simulink model "MultiSiteCoherenceTriggerDetector"  (R2016b)
settings: Solver=FixedStepDiscrete  StartTime=0.0  StopTime=inf  FixedStep=sCoreParams.core.stepPeriod  RelTol=1e-3
undefined symbols (not defined in the file): Low, sCoreParams, sCoreParams_decoders_txDetector_anyAll, sCoreParams_decoders_txDetector_detectChannelInds, sCoreParams_decoders_txDetector_nDetectionsRequested, sCoreParams_decoders_txDetector_ProbabilityOfStim, sCoreParams_decoders_txDetector_txRMS, sCoreParams_decoders_txDetector_txRMSLower, sCoreParams_decoders_txDetector_txSign, sCoreParams_stimulator_possibleStimRealChannelNumbers
libraries: simulink x3, dspswit3 x3, dspsigops x1
settings Model: DataTypeOverride=Double  MinMaxOverflowLogging=ForceOff  ParamWorkspaceSource=ReferencedWorkspace  Creator=anish  LastModifiedBy=rzelmann
settings SolverCC: EnableConcurrentExecution=on
settings DataIOCC: SaveFormat=StructureWithTime  SignalLoggingSaveFormat=ModelDataLogs  SaveOutput=off  SignalLogging=off  DSMLogging=off  SaveTime=off
settings OptimizationCC: BlockReduction=off  ConditionallyExecuteInputs=off  DefaultParameterBehavior=Inlined  OptimizeBlockIOStorage=off  BufferReuse=off  GlobalBufferReuse=off  ExpressionFolding=off  LocalBlockOutputs=off  LifeSpan=inf
settings DebuggingCC: SignalRangeChecking=error  SaveWithParameterizedLinksMsg=none  MultiTaskDSMMsg=warning  MultiTaskCondExecSysMsg=none  AllowSymbolicDim=off  ModelReferenceSymbolNameMessage=none  StateNameClashWarn=warning  SFUnexpectedBacktrackingDiag=warning  SFNoUnconditionalDefaultTransitionDiag=warning  SFExecutionAtInitializationDiag=none
settings HardwareCC: ProdBitPerPointer=32  ProdBitPerSizeT=32  ProdBitPerPtrDiffT=32  ProdLargestAtomicFloat=None  ProdWordSize=32  ProdLongLongMode=on  ProdHWDeviceType=Generic->32-bit x86 compatible  TargetBitPerPointer=64  TargetLargestAtomicFloat=Float  TargetLongLongMode=on  TargetIntDivRoundTo=Zero  TargetEndianess=LittleEndian  TargetWordSize=64  TargetHWDeviceType=Intel->x86-64 (Windows64)
settings ModelReferenceCC: ModelReferenceNumInstancesAllowed=Single  ModelReferencePassRootInputsByReference=off
settings RTWCC: SystemTargetFile=slrt.tlc  TemplateMakefile=slrt_default_tmf  Description=Simulink Real-Time  BuildConfiguration=Faster Runs  RTWCompilerOptimization=on
settings ConfigComp: CovMetricSettings=dw  CovHtmlReporting=on  CovSaveCumulativeToWorkspaceVar=on  CovSaveSingleToWorkspaceVar=on  CovExternalEMLEnable=off  CovSFcnEnable=off

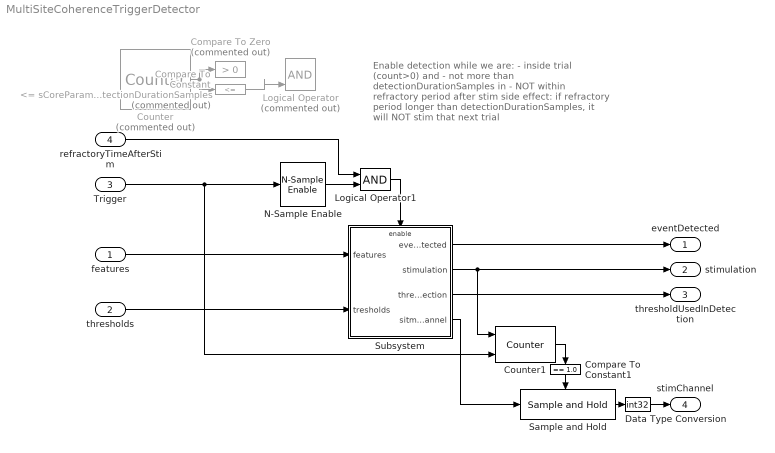
== system MultiSiteCoherenceTriggerDetector ==
  note: Enable detection while we are:
      |  -  inside trial (count>0) and
      | - not more than detectionDurationSamples in
      | - NOT within refractory period after stim
      | side effect: if refractory period longer than detectionDurationSamples, it will NOT stim that next trial
  features : Inport  PortDimensions=[1 sCoreParams.decoders.txDetector.nPairs]  SampleTime=sCoreParams.core.stepPeriod
  thresholds : Inport  Port=2  PortDimensions=[1 sCoreParams.decoders.txDetector.nPairs]  SampleTime=sCoreParams.core.stepPeriod
  Trigger : Inport  Port=3  OutDataTypeStr=int32
  refractoryTimeAfterStim : Inport  Port=4  OutDataTypeStr=boolean  SampleTime=sCoreParams.core.stepPeriod
  Compare To Constant : simulink/Logic and Bit Operations/Compare To Constant  Commented=on  relop=<=  const=sCoreParams.decoders.txDetector.detectionDurationSamples  OutDataTypeStr=boolean
  Compare To Constant1 : simulink/Logic and Bit Operations/Compare To Constant  relop===  const=1.0  OutDataTypeStr=boolean
  Compare To Zero : simulink/Logic and Bit Operations/Compare To Zero  Commented=on  relop=>  OutDataTypeStr=boolean
  Counter : dspswit3/Counter  Commented=on  Direction=Up  CountEvent=Free running  CounterSize=16 bits  MaxCount=255  InitialCount=0  Output=Count  HitValue=sCoreParams.decoders.txDetector.detectionDurationSamples  ResetInput=on  SamplesPerFrame=1  Ts=sCoreParams.core.stepPeriod  CntDtype=int32  HitDtype=Logical
  Counter1 : dspswit3/Counter  Direction=Up  CountEvent=Rising edge  CounterSize=User defined  MaxCount=1024  InitialCount=0  Output=Count  HitValue=1  ResetInput=on  SamplesPerFrame=1  Ts=1  CntDtype=double  HitDtype=Logical
  Data Type Conversion : DataTypeConversion  OutDataTypeStr=int32
  Logical Operator : Logic  Commented=on  IconShape=distinctive  AllPortsSameDT=off  OutDataTypeStr=boolean
  Logical Operator1 : Logic  IconShape=distinctive  AllPortsSameDT=off  OutDataTypeStr=boolean
  N-Sample Enable : dspswit3/N-Sample Enable  N=sCoreParams.decoders.txDetector.detectionDurationSamples  ActiveLevel=Low (0)  reset=on  TriggerType=Non-zero sample  Ts=1  DataType=Logical
  Sample and Hold : dspsigops/Sample and Hold  trig=Rising edge  initCond=0  latchinput=off
  Subsystem : Subsystem
  eventDetected : Outport  SampleTime=sCoreParams.core.stepPeriod
  stimulation : Outport  Port=2  SampleTime=sCoreParams.core.stepPeriod
  thresholdUsedInDetection : Outport  Port=3  SampleTime=sCoreParams.core.stepPeriod
  stimChannel : Outport  Port=4  OutDataTypeStr=int32
  wires:
  features/1 -> Subsystem/1(features)
  thresholds/1 -> Subsystem/2(tresholds)
  Subsystem/1(eventDetected) -> eventDetected/1
  Subsystem/2(stimulation) -> stimulation/1, Counter1/1
  Subsystem/3(thresholdUsedInDetection) -> thresholdUsedInDetection/1
  Trigger/1 -> Counter1/2, N-Sample Enable/1
  Logical Operator1/1 -> Subsystem/Enable
  Subsystem/4(sitmChannel) -> Sample and Hold/1
  Data Type Conversion/1 -> stimChannel/1
  Counter/1 -> Compare To Constant/1, Compare To Zero/1
  Compare To Constant/1 -> Logical Operator/2
  Sample and Hold/1 -> Data Type Conversion/1
  Counter1/1 -> Compare To Constant1/1
  refractoryTimeAfterStim/1 -> Logical Operator1/1
  N-Sample Enable/1 -> Logical Operator1/2
  Compare To Constant1/1 -> Sample and Hold/Trigger

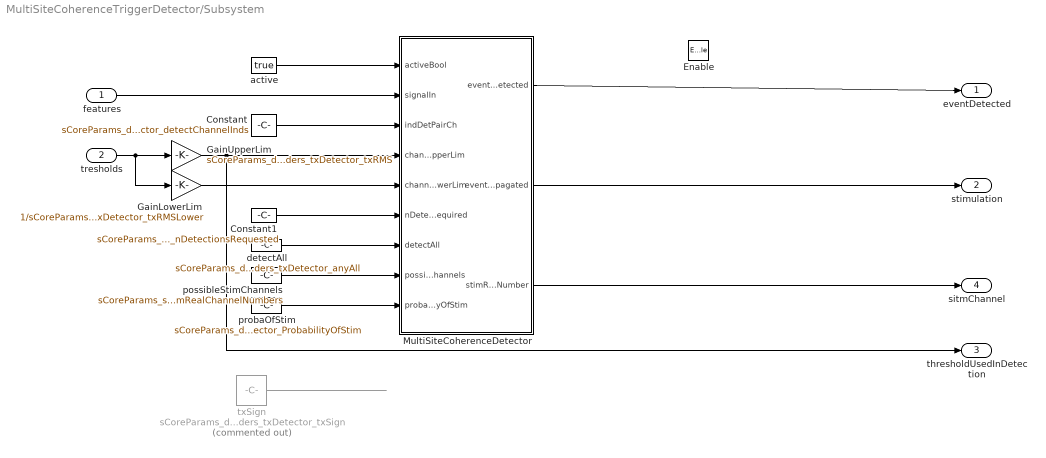
== system MultiSiteCoherenceTriggerDetector/Subsystem ==
  features : Inport
  tresholds : Inport  Port=2
  Enable : EnablePort
  Constant : Constant  Value=sCoreParams_decoders_txDetector_detectChannelInds  SampleTime=Inf
  Constant1 : Constant  Value=sCoreParams_decoders_txDetector_nDetectionsRequested  SampleTime=Inf
  GainLowerLim : Gain  Gain=1/sCoreParams_decoders_txDetector_txRMSLower
  GainUpperLim : Gain  Gain=sCoreParams_decoders_txDetector_txRMS
  MultiSiteCoherenceDetector : MATLAB Function  TreatAsAtomicUnit=on
  active : Constant  Value=true
  detectAll : Constant  Value=sCoreParams_decoders_txDetector_anyAll
  possibleStimChannels : Constant  Value=sCoreParams_stimulator_possibleStimRealChannelNumbers
  probaOfStim : Constant  Value=sCoreParams_decoders_txDetector_ProbabilityOfStim
  txSign : Constant  Commented=on  Value=sCoreParams_decoders_txDetector_txSign
  eventDetected : Outport
  stimulation : Outport  Port=2
  thresholdUsedInDetection : Outport  Port=3
  sitmChannel : Outport  Port=4
  wires:
  GainUpperLim/1 -> thresholdUsedInDetection/1, MultiSiteCoherenceDetector/4(channelThresholdUpperLim)
  MultiSiteCoherenceDetector/2(eventPropagated) -> stimulation/1
  Constant/1 -> MultiSiteCoherenceDetector/3(indDetPairCh)
  Constant1/1 -> MultiSiteCoherenceDetector/6(nDetectionsRequired)
  active/1 -> MultiSiteCoherenceDetector/1(activeBool)
  txSign/1 -> ?
  features/1 -> MultiSiteCoherenceDetector/2(signalIn)
  MultiSiteCoherenceDetector/1(eventDetected) -> eventDetected/1
  tresholds/1 -> GainLowerLim/1, GainUpperLim/1
  detectAll/1 -> MultiSiteCoherenceDetector/7(detectAll)
  MultiSiteCoherenceDetector/3(stimRealChannelNumber) -> sitmChannel/1
  GainLowerLim/1 -> MultiSiteCoherenceDetector/5(channelThresholdLowerLim)
  possibleStimChannels/1 -> MultiSiteCoherenceDetector/8(possibleStimChannels)
  probaOfStim/1 -> MultiSiteCoherenceDetector/9(probabilityOfStim)

== matlab function MultiSiteCoherenceTriggerDetector/Subsystem/MultiSiteCoherenceDetector ==
  data: activeBool input; eventDetected output; signalIn input; indDetPairCh input; channelThresholdUpperLim input; channelThresholdLowerLim input; nDetectionsRequired input; eventPropagated output; detectAll input; stimRealChannelNumber output; possibleStimChannels input; probabilityOfStim input
function [eventDetected, eventPropagated, stimRealChannelNumber] = MultiSiteCoherenceDetector(activeBool, signalIn, indDetPairCh, channelThresholdUpperLim, channelThresholdLowerLim, nDetectionsRequired, detectAll, possibleStimChannels, probabilityOfStim)
%#codegen

if (detectAll >= 1) % 1 means ALL - 0 means ANY
    [eventDetected, eventPropagated, stimRealChannelNumber] = MultiSiteCoherenceDetectorAll_EML(activeBool, signalIn, indDetPairCh, channelThresholdUpperLim, channelThresholdLowerLim, nDetectionsRequired, possibleStimChannels, probabilityOfStim);
else
    [eventDetected, eventPropagated, stimRealChannelNumber] = MultiSiteCoherenceDetectorAny_EML(activeBool, signalIn, indDetPairCh, channelThresholdUpperLim, channelThresholdLowerLim, nDetectionsRequired, possibleStimChannels, probabilityOfStim);
end
